simulink model "JX_Kinect_multi"  (Simulink 7.7)
settings: Solver=ode4  StartTime=0.0  StopTime=inf  FixedStep=sample_time  RelTol=1e-3
InitFcn:
  | sample_time=0.005;%0.004;%0.0025;%0.02;
  | DeltaT = 0.02;
  | g = 9.81;
  | H0 = g%0.3165;
  | Kl = 1;
  | 
  | Omega_r = 1.6;%for Horizontal reference
  | Zeta_r = 1; %for Horizontal reference
  | Omega = 1.8;%for Horizontal Control
  | Zeta = 0.5;    %for Horizontal Control
  | 
  | Omega_h_r = 2.5; %for vertical reference
  | Zeta_h_r = 0.8;  %for vertical reference
  | Omega_h = 2.7;    %for vertical control
  | Zeta_h = 0.8;         %for vertical control
  | PI=pi;
  | 
  | Mass = 1.15;
  | Acc_Max = 4;
  | Acc_Max_h = 4;
  | 
  | Max_RP = 60;
  | 
  | % for NN
  | n = 5;
  | r = 3;
  | n2 = 5;
  | NN_ST = 0.02;
  | 
  | GAMA_V = 6;
  | gama_V_e = 0.01;
  | 
  | GAMA_W = GAMA_V;
  | gama_W_e =0.01;
  | 
  | % deadzone
  | NN_Deadzone_Z = 0;
  | 
  | % inputs nomalizaton parameters
  | NN_Z_y_min = -3;
  | NN_Z_y_max = 0.5;
  | 
  | NN_Z_v_max = 8;
  | NN_Z_v_min = -NN_Z_v_max;
  | 
  | % alpha = 0.034;
  | alpha = 1;
  | % c_f = 0.0015;
  | c_f = 0.001;
  | c_y_tilt = 1*0.5;
  | 
  | %for WK paras
  | Heightcontrol = 0.08;
  | Scale_Factor=1;
  | yoffset=0;
  | 
  | load MaoBi_Oct04_2_int.mat
  | MB_Interp.time = [];
undefined symbols (not defined in the file or in its folder): DiscIntNeverNeededParam
libraries: simulink x14, dspadpt3 x6, X330_Control x4, nid_lib x2
(part 3 of 4)

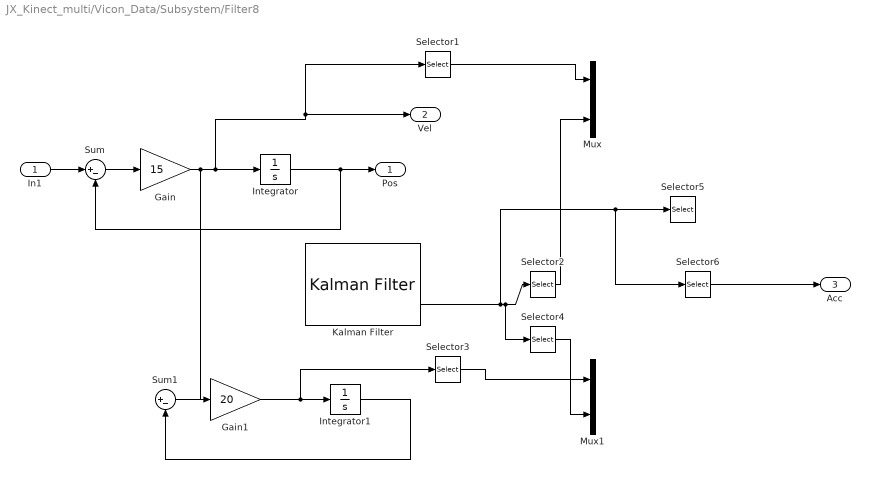
== system JX_Kinect_multi/Vicon_Data/Subsystem/Filter8 ==
  In1 : Inport
  Gain : Gain  Gain=15
  Gain1 : Gain  Gain=20
  Integrator : Integrator
  Integrator1 : Integrator
  Kalman Filter : dspadpt3/Kalman Filter  SystemSampleTime=-1  num_targets=1  sourceEnable=Always  isReset=on  X=zeros([9, 1])  P=zeros(9)  A=[1 sample_time sample_time*sample_time/2 zeros(1,6);0 1 sample_time zeros(1,6);0 0 1 zeros(1,6);0 0 0 1 sample_time sample_time*sample_time/2 0 0 0;zeros(1,4) 1 sample_time zeros(1,3);zeros(1,5) 1 zeros(1,3);zeros(1,6) 1 sample_time sample_time*sample_time/2;zeros(1,7) 1 sample_time;zeros(1,8) 1]  sourceMeasure=Specify via Dialog  H=[1 zeros(1,8); zeros(1,3) 1 zeros(1,5);zeros(1,6) 1 0 0]  Q=diag([0 0.001 0.001 0 0.001 0.001 0 0.001 0.001])  R=0.001*eye(3)  isOutputEstMeasure=on  isOutputEstState=on  isOutputEstError=off  isOutputPrdMeasure=off  isOutputPrdState=off  isOutputPrdError=off
  Mux : Mux  Inputs=2
  Mux1 : Mux  Inputs=2
  Selector1 : Selector  InputPortWidth=3  IndexOptions=Index vector (dialog)  Indices=[2]  OutputSizes=1
  Selector2 : Selector  InputPortWidth=9  IndexOptions=Index vector (dialog)  Indices=[5]  OutputSizes=1
  Selector3 : Selector  InputPortWidth=3  IndexOptions=Index vector (dialog)  Indices=[2]  OutputSizes=1
  Selector4 : Selector  InputPortWidth=9  IndexOptions=Index vector (dialog)  Indices=[6]  OutputSizes=1
  Selector5 : Selector  InputPortWidth=9  IndexOptions=Index vector (dialog)  Indices=[2 5 8]  OutputSizes=1
  Selector6 : Selector  InputPortWidth=9  IndexOptions=Index vector (dialog)  Indices=[3 6 9]  OutputSizes=1
  Sum : Sum  Inputs=|+-
  Sum1 : Sum  Inputs=|+-
  Pos : Outport
  Vel : Outport  Port=2
  Acc : Outport  Port=3
  wires:
  Selector6/1 -> Acc/1
  Selector4/1 -> Mux1/2
  Selector3/1 -> Mux1/1
  Selector2/1 -> Mux/2
  Integrator1/1 -> Sum1/2
  Gain1/1 -> Selector3/1, Integrator1/1
  Sum1/1 -> Gain1/1
  Kalman Filter/2 -> Selector6/1, Selector5/1, Selector2/1, Selector4/1
  Selector1/1 -> Mux/1
  In1/1 -> Sum/1
  Integrator/1 -> Sum/2, Pos/1
  Gain/1 -> Sum1/1, Vel/1, Selector1/1, Integrator/1
  Sum/1 -> Gain/1

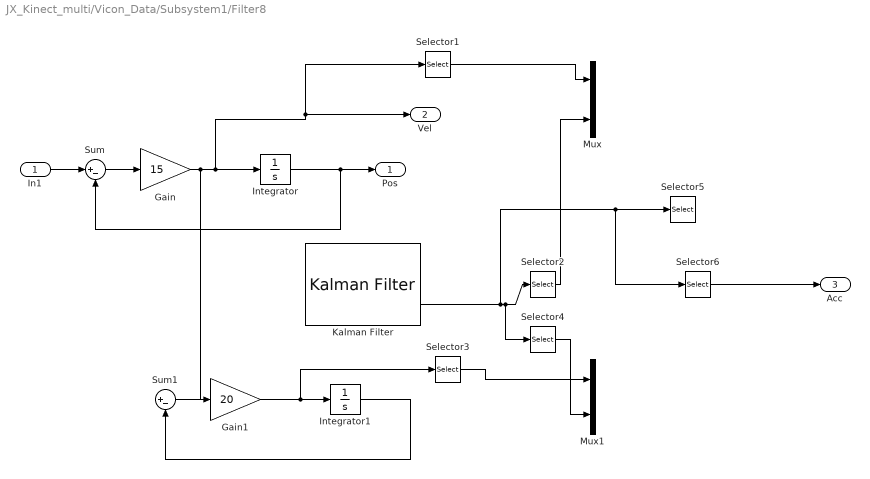
== system JX_Kinect_multi/Vicon_Data/Subsystem1/Filter8 ==
  In1 : Inport
  Gain : Gain  Gain=15
  Gain1 : Gain  Gain=20
  Integrator : Integrator
  Integrator1 : Integrator
  Kalman Filter : dspadpt3/Kalman Filter  SystemSampleTime=-1  num_targets=1  sourceEnable=Always  isReset=on  X=zeros([9, 1])  P=zeros(9)  A=[1 sample_time sample_time*sample_time/2 zeros(1,6);0 1 sample_time zeros(1,6);0 0 1 zeros(1,6);0 0 0 1 sample_time sample_time*sample_time/2 0 0 0;zeros(1,4) 1 sample_time zeros(1,3);zeros(1,5) 1 zeros(1,3);zeros(1,6) 1 sample_time sample_time*sample_time/2;zeros(1,7) 1 sample_time;zeros(1,8) 1]  sourceMeasure=Specify via Dialog  H=[1 zeros(1,8); zeros(1,3) 1 zeros(1,5);zeros(1,6) 1 0 0]  Q=diag([0 0.001 0.001 0 0.001 0.001 0 0.001 0.001])  R=0.001*eye(3)  isOutputEstMeasure=on  isOutputEstState=on  isOutputEstError=off  isOutputPrdMeasure=off  isOutputPrdState=off  isOutputPrdError=off
  Mux : Mux  Inputs=2
  Mux1 : Mux  Inputs=2
  Selector1 : Selector  InputPortWidth=3  IndexOptions=Index vector (dialog)  Indices=[2]  OutputSizes=1
  Selector2 : Selector  InputPortWidth=9  IndexOptions=Index vector (dialog)  Indices=[5]  OutputSizes=1
  Selector3 : Selector  InputPortWidth=3  IndexOptions=Index vector (dialog)  Indices=[2]  OutputSizes=1
  Selector4 : Selector  InputPortWidth=9  IndexOptions=Index vector (dialog)  Indices=[6]  OutputSizes=1
  Selector5 : Selector  InputPortWidth=9  IndexOptions=Index vector (dialog)  Indices=[2 5 8]  OutputSizes=1
  Selector6 : Selector  InputPortWidth=9  IndexOptions=Index vector (dialog)  Indices=[3 6 9]  OutputSizes=1
  Sum : Sum  Inputs=|+-
  Sum1 : Sum  Inputs=|+-
  Pos : Outport
  Vel : Outport  Port=2
  Acc : Outport  Port=3
  wires:
  Selector6/1 -> Acc/1
  Selector4/1 -> Mux1/2
  Selector3/1 -> Mux1/1
  Selector2/1 -> Mux/2
  Integrator1/1 -> Sum1/2
  Gain1/1 -> Selector3/1, Integrator1/1
  Sum1/1 -> Gain1/1
  Kalman Filter/2 -> Selector6/1, Selector5/1, Selector2/1, Selector4/1
  Selector1/1 -> Mux/1
  In1/1 -> Sum/1
  Integrator/1 -> Sum/2, Pos/1
  Gain/1 -> Sum1/1, Vel/1, Selector1/1, Integrator/1
  Sum/1 -> Gain/1

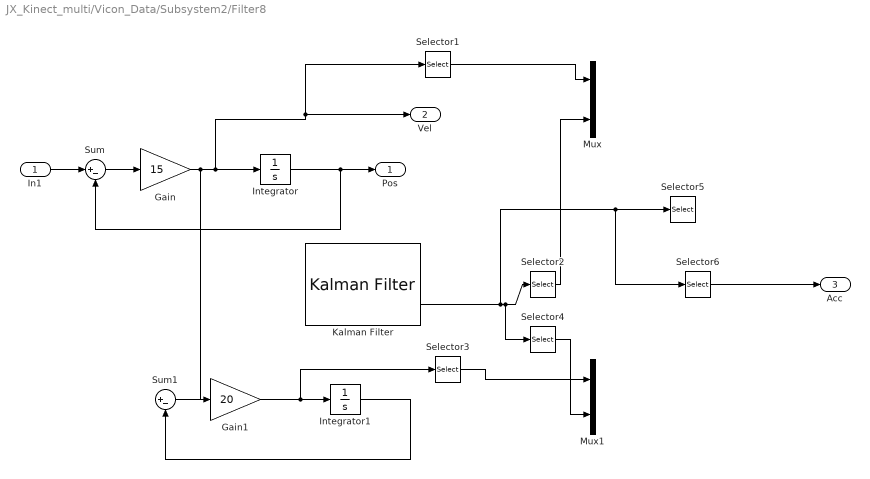
== system JX_Kinect_multi/Vicon_Data/Subsystem2/Filter8 ==
  In1 : Inport
  Gain : Gain  Gain=15
  Gain1 : Gain  Gain=20
  Integrator : Integrator
  Integrator1 : Integrator
  Kalman Filter : dspadpt3/Kalman Filter  SystemSampleTime=-1  num_targets=1  sourceEnable=Always  isReset=on  X=zeros([9, 1])  P=zeros(9)  A=[1 sample_time sample_time*sample_time/2 zeros(1,6);0 1 sample_time zeros(1,6);0 0 1 zeros(1,6);0 0 0 1 sample_time sample_time*sample_time/2 0 0 0;zeros(1,4) 1 sample_time zeros(1,3);zeros(1,5) 1 zeros(1,3);zeros(1,6) 1 sample_time sample_time*sample_time/2;zeros(1,7) 1 sample_time;zeros(1,8) 1]  sourceMeasure=Specify via Dialog  H=[1 zeros(1,8); zeros(1,3) 1 zeros(1,5);zeros(1,6) 1 0 0]  Q=diag([0 0.001 0.001 0 0.001 0.001 0 0.001 0.001])  R=0.001*eye(3)  isOutputEstMeasure=on  isOutputEstState=on  isOutputEstError=off  isOutputPrdMeasure=off  isOutputPrdState=off  isOutputPrdError=off
  Mux : Mux  Inputs=2
  Mux1 : Mux  Inputs=2
  Selector1 : Selector  InputPortWidth=3  IndexOptions=Index vector (dialog)  Indices=[2]  OutputSizes=1
  Selector2 : Selector  InputPortWidth=9  IndexOptions=Index vector (dialog)  Indices=[5]  OutputSizes=1
  Selector3 : Selector  InputPortWidth=3  IndexOptions=Index vector (dialog)  Indices=[2]  OutputSizes=1
  Selector4 : Selector  InputPortWidth=9  IndexOptions=Index vector (dialog)  Indices=[6]  OutputSizes=1
  Selector5 : Selector  InputPortWidth=9  IndexOptions=Index vector (dialog)  Indices=[2 5 8]  OutputSizes=1
  Selector6 : Selector  InputPortWidth=9  IndexOptions=Index vector (dialog)  Indices=[3 6 9]  OutputSizes=1
  Sum : Sum  Inputs=|+-
  Sum1 : Sum  Inputs=|+-
  Pos : Outport
  Vel : Outport  Port=2
  Acc : Outport  Port=3
  wires:
  Selector6/1 -> Acc/1
  Selector4/1 -> Mux1/2
  Selector3/1 -> Mux1/1
  Selector2/1 -> Mux/2
  Integrator1/1 -> Sum1/2
  Gain1/1 -> Selector3/1, Integrator1/1
  Sum1/1 -> Gain1/1
  Kalman Filter/2 -> Selector6/1, Selector5/1, Selector2/1, Selector4/1
  Selector1/1 -> Mux/1
  In1/1 -> Sum/1
  Integrator/1 -> Sum/2, Pos/1
  Gain/1 -> Sum1/1, Vel/1, Selector1/1, Integrator/1
  Sum/1 -> Gain/1

== system JX_Kinect_multi/Vicon_Data/Vicon Filter/Filter7 ==
  In1 : Inport
  Kalman Filter : dspadpt3/Kalman Filter  SystemSampleTime=-1  num_targets=1  sourceEnable=Always  isReset=on  X=zeros([12, 1])  P=zeros(12)  A=[1 sample_time sample_time*sample_time/2 zeros(1,9);0 1 sample_time zeros(1,9);0 0 1 zeros(1,9);0 0 0 1 sample_time sample_time*sample_time/2 zeros(1,6);zeros(1,4) 1 sample_time zeros(1,6);zeros(1,5) 1 zeros(1,6);zeros(1,6) 1 sample_time sample_time*sample_time/2 zeros(1,3);zeros(1,7) 1 sample_time zeros(1,3);zeros(1,8) 1 zeros(1,3);zeros(1,9) 1 sample_time sample_time*sample_time/2;zeros(1,10) 1 sample_time;zeros(1,11) 1];  sourceMeasure=Specify via Dialog  H=[1 zeros(1,11); zeros(1,3) 1 zeros(1,8);zeros(1,6) 1 zeros(1,5);zeros(1,9) 1 0 0]  Q=diag([0 0.001 0.001 0 0.001 0.001 0 0.001 0.001 0 0.001 0.001]);  R=diag([0.001 0.001 0.001 0.05])  isOutputEstMeasure=off  isOutputEstState=on  isOutputEstError=off  isOutputPrdMeasure=off  isOutputPrdState=off  isOutputPrdError=off
  Selector1 : Selector  InputPortWidth=12  IndexOptions=Index vector (dialog)  Indices=[10]  OutputSizes=1
  Selector5 : Selector  InputPortWidth=12  IndexOptions=Index vector (dialog)  Indices=[2 5 8]  OutputSizes=1
  Selector6 : Selector  InputPortWidth=12  IndexOptions=Index vector (dialog)  Indices=[3 6 9]  OutputSizes=1
  Vel : Outport
  Acc : Outport  Port=2
  Psi : Outport  Port=3
  wires:
  Selector1/1 -> Psi/1
  Selector5/1 -> Vel/1
  In1/1 -> Kalman Filter/1
  Kalman Filter/1 -> Selector1/1, Selector5/1, Selector6/1
  Selector6/1 -> Acc/1

== system JX_Kinect_multi/Vicon_Data/Vicon Filter1/Filter7 ==
  In1 : Inport
  Kalman Filter : dspadpt3/Kalman Filter  SystemSampleTime=-1  num_targets=1  sourceEnable=Always  isReset=on  X=zeros([12, 1])  P=zeros(12)  A=[1 sample_time sample_time*sample_time/2 zeros(1,9);0 1 sample_time zeros(1,9);0 0 1 zeros(1,9);0 0 0 1 sample_time sample_time*sample_time/2 zeros(1,6);zeros(1,4) 1 sample_time zeros(1,6);zeros(1,5) 1 zeros(1,6);zeros(1,6) 1 sample_time sample_time*sample_time/2 zeros(1,3);zeros(1,7) 1 sample_time zeros(1,3);zeros(1,8) 1 zeros(1,3);zeros(1,9) 1 sample_time sample_time*sample_time/2;zeros(1,10) 1 sample_time;zeros(1,11) 1];  sourceMeasure=Specify via Dialog  H=[1 zeros(1,11); zeros(1,3) 1 zeros(1,8);zeros(1,6) 1 zeros(1,5);zeros(1,9) 1 0 0]  Q=diag([0 0.001 0.001 0 0.001 0.001 0 0.001 0.001 0 0.001 0.001]);  R=diag([0.001 0.001 0.001 0.05])  isOutputEstMeasure=off  isOutputEstState=on  isOutputEstError=off  isOutputPrdMeasure=off  isOutputPrdState=off  isOutputPrdError=off
  Selector1 : Selector  InputPortWidth=12  IndexOptions=Index vector (dialog)  Indices=[10]  OutputSizes=1
  Selector5 : Selector  InputPortWidth=12  IndexOptions=Index vector (dialog)  Indices=[2 5 8]  OutputSizes=1
  Selector6 : Selector  InputPortWidth=12  IndexOptions=Index vector (dialog)  Indices=[3 6 9]  OutputSizes=1
  Vel : Outport
  Acc : Outport  Port=2
  Psi : Outport  Port=3
  wires:
  Selector1/1 -> Psi/1
  Selector5/1 -> Vel/1
  In1/1 -> Kalman Filter/1
  Kalman Filter/1 -> Selector1/1, Selector5/1, Selector6/1
  Selector6/1 -> Acc/1

== system JX_Kinect_multi/Vicon_Data/Vicon Filter2/Filter7 ==
  In1 : Inport
  Kalman Filter : dspadpt3/Kalman Filter  SystemSampleTime=-1  num_targets=1  sourceEnable=Always  isReset=on  X=zeros([12, 1])  P=zeros(12)  A=[1 sample_time sample_time*sample_time/2 zeros(1,9);0 1 sample_time zeros(1,9);0 0 1 zeros(1,9);0 0 0 1 sample_time sample_time*sample_time/2 zeros(1,6);zeros(1,4) 1 sample_time zeros(1,6);zeros(1,5) 1 zeros(1,6);zeros(1,6) 1 sample_time sample_time*sample_time/2 zeros(1,3);zeros(1,7) 1 sample_time zeros(1,3);zeros(1,8) 1 zeros(1,3);zeros(1,9) 1 sample_time sample_time*sample_time/2;zeros(1,10) 1 sample_time;zeros(1,11) 1];  sourceMeasure=Specify via Dialog  H=[1 zeros(1,11); zeros(1,3) 1 zeros(1,8);zeros(1,6) 1 zeros(1,5);zeros(1,9) 1 0 0]  Q=diag([0 0.001 0.001 0 0.001 0.001 0 0.001 0.001 0 0.001 0.001]);  R=diag([0.001 0.001 0.001 0.05])  isOutputEstMeasure=off  isOutputEstState=on  isOutputEstError=off  isOutputPrdMeasure=off  isOutputPrdState=off  isOutputPrdError=off
  Selector1 : Selector  InputPortWidth=12  IndexOptions=Index vector (dialog)  Indices=[10]  OutputSizes=1
  Selector5 : Selector  InputPortWidth=12  IndexOptions=Index vector (dialog)  Indices=[2 5 8]  OutputSizes=1
  Selector6 : Selector  InputPortWidth=12  IndexOptions=Index vector (dialog)  Indices=[3 6 9]  OutputSizes=1
  Vel : Outport
  Acc : Outport  Port=2
  Psi : Outport  Port=3
  wires:
  Selector1/1 -> Psi/1
  Selector5/1 -> Vel/1
  In1/1 -> Kalman Filter/1
  Kalman Filter/1 -> Selector1/1, Selector5/1, Selector6/1
  Selector6/1 -> Acc/1

== system JX_Kinect_multi/Kinect/Subsystem/Front or Center or Back/If Back ==
  In1 : Inport
  Action Port : ActionPort  ActionType=else
  Out1 : Outport
  wires:
  In1/1 -> Out1/1

== system JX_Kinect_multi/Kinect/Subsystem/Front or Center or Back/If Center ==
  In1 : Inport
  Action Port : ActionPort  ActionType=elseif
  Out1 : Outport
  wires:
  In1/1 -> Out1/1

== system JX_Kinect_multi/Kinect/Subsystem/Front or Center or Back/If front ==
  In1 : Inport
  Action Port : ActionPort  ActionType=then
  Out1 : Outport
  wires:
  In1/1 -> Out1/1

== system JX_Kinect_multi/Kinect/Subsystem/Up or Center or Down/Center ==
  In1 : Inport
  Action Port : ActionPort  ActionType=elseif
  Out1 : Outport
  wires:
  In1/1 -> Out1/1

== system JX_Kinect_multi/Kinect/Subsystem/Up or Center or Down/Down max ==
  In1 : Inport
  Action Port : ActionPort  ActionType=else
  Out1 : Outport
  wires:
  In1/1 -> Out1/1

== system JX_Kinect_multi/Kinect/Subsystem/Up or Center or Down/Down1 ==
  In1 : Inport
  Action Port : ActionPort  ActionType=elseif
  Out1 : Outport
  wires:
  In1/1 -> Out1/1

== system JX_Kinect_multi/Kinect/Subsystem/Up or Center or Down/Top1 ==
  In1 : Inport
  Action Port : ActionPort  ActionType=then
  Out1 : Outport
  wires:
  In1/1 -> Out1/1

== system JX_Kinect_multi/Kinect/Subsystem1/Up or Center or Down/Center ==
  In1 : Inport
  Action Port : ActionPort  ActionType=elseif
  Out1 : Outport
  wires:
  In1/1 -> Out1/1

== system JX_Kinect_multi/Kinect/Subsystem1/Up or Center or Down/Down1 ==
  In1 : Inport
  Action Port : ActionPort  ActionType=else
  Out1 : Outport
  wires:
  In1/1 -> Out1/1

== system JX_Kinect_multi/Kinect/Subsystem1/Up or Center or Down/Top1 ==
  In1 : Inport
  Action Port : ActionPort  ActionType=then
  Out1 : Outport
  wires:
  In1/1 -> Out1/1

== system JX_Kinect_multi/Vicon_Data/Raw Quad Pose from Vicon/Process Vicon Raw Data1/Flip_pi1 ==
  Angle : Inport
  Add : Sum  Inputs=-+
  Compare To Constant1 : simulink/Logic and Bit Operations/Compare To Constant  SystemSampleTime=-1  relop=>  const=pi  LogicOutDataTypeMode=uint8  ZeroCross=off
  Constant : Constant  Value=2*pi
  Data Type Duplicate : DataTypeDuplicate
  Flip_0_to_2pi : Subsystem
      mask Type: Flip zero to 2pi
      mask Description: Flips the inputs into the range zero to +2pi
      mask Help: Flips the inputs into the range zero to +2pi
      mask Display: disp('Flip_0_2pi')
  Switch : Switch  Criteria=u2 ~= 0
  Angle_Flip : Outport
  wires:
  Angle/1 -> Flip_0_to_2pi/1(Angle), Data Type Duplicate/2
  Flip_0_to_2pi/1(Angle_Flip) -> Switch/3, Compare To Constant1/1, Add/2
  Compare To Constant1/1 -> Switch/2
  Constant/1 -> Add/1
  Add/1 -> Switch/1
  Switch/1 -> Angle_Flip/1, Data Type Duplicate/1

== system JX_Kinect_multi/Vicon_Data/Raw Quad Pose from Vicon/Process Vicon Raw Data2/Flip_pi1 ==
  Angle : Inport
  Add : Sum  Inputs=-+
  Compare To Constant1 : simulink/Logic and Bit Operations/Compare To Constant  SystemSampleTime=-1  relop=>  const=pi  LogicOutDataTypeMode=uint8  ZeroCross=off
  Constant : Constant  Value=2*pi
  Data Type Duplicate : DataTypeDuplicate
  Flip_0_to_2pi : Subsystem
      mask Type: Flip zero to 2pi
      mask Description: Flips the inputs into the range zero to +2pi
      mask Help: Flips the inputs into the range zero to +2pi
      mask Display: disp('Flip_0_2pi')
  Switch : Switch  Criteria=u2 ~= 0
  Angle_Flip : Outport
  wires:
  Switch/1 -> Data Type Duplicate/1, Angle_Flip/1
  Add/1 -> Switch/1
  Constant/1 -> Add/1
  Compare To Constant1/1 -> Switch/2
  Flip_0_to_2pi/1(Angle_Flip) -> Add/2, Compare To Constant1/1, Switch/3
  Angle/1 -> Data Type Duplicate/2, Flip_0_to_2pi/1(Angle)

== system JX_Kinect_multi/Vicon_Data/Raw Quad Pose from Vicon/Process Vicon Raw Data3/Flip_pi1 ==
  Angle : Inport
  Add : Sum  Inputs=-+
  Compare To Constant1 : simulink/Logic and Bit Operations/Compare To Constant  SystemSampleTime=-1  relop=>  const=pi  LogicOutDataTypeMode=uint8  ZeroCross=off
  Constant : Constant  Value=2*pi
  Data Type Duplicate : DataTypeDuplicate
  Flip_0_to_2pi : Subsystem
      mask Type: Flip zero to 2pi
      mask Description: Flips the inputs into the range zero to +2pi
      mask Help: Flips the inputs into the range zero to +2pi
      mask Display: disp('Flip_0_2pi')
  Switch : Switch  Criteria=u2 ~= 0
  Angle_Flip : Outport
  wires:
  Angle/1 -> Flip_0_to_2pi/1(Angle), Data Type Duplicate/2
  Flip_0_to_2pi/1(Angle_Flip) -> Switch/3, Compare To Constant1/1, Add/2
  Compare To Constant1/1 -> Switch/2
  Constant/1 -> Add/1
  Add/1 -> Switch/1
  Switch/1 -> Angle_Flip/1, Data Type Duplicate/1

== system JX_Kinect_multi/Vicon_Data/Raw Quad Pose from Vicon/Process Vicon Raw Data4/Flip_pi1 ==
  Angle : Inport
  Add : Sum  Inputs=-+
  Compare To Constant1 : simulink/Logic and Bit Operations/Compare To Constant  SystemSampleTime=-1  relop=>  const=pi  LogicOutDataTypeMode=uint8  ZeroCross=off
  Constant : Constant  Value=2*pi
  Data Type Duplicate : DataTypeDuplicate
  Flip_0_to_2pi : Subsystem
      mask Type: Flip zero to 2pi
      mask Description: Flips the inputs into the range zero to +2pi
      mask Help: Flips the inputs into the range zero to +2pi
      mask Display: disp('Flip_0_2pi')
  Switch : Switch  Criteria=u2 ~= 0
  Angle_Flip : Outport
  wires:
  Switch/1 -> Data Type Duplicate/1, Angle_Flip/1
  Add/1 -> Switch/1
  Constant/1 -> Add/1
  Compare To Constant1/1 -> Switch/2
  Flip_0_to_2pi/1(Angle_Flip) -> Add/2, Compare To Constant1/1, Switch/3
  Angle/1 -> Data Type Duplicate/2, Flip_0_to_2pi/1(Angle)

== system JX_Kinect_multi/Vicon_Data/Raw Quad Pose from Vicon/Process Vicon Raw Data6/Flip_pi1 ==
  Angle : Inport
  Add : Sum  Inputs=-+
  Compare To Constant1 : simulink/Logic and Bit Operations/Compare To Constant  SystemSampleTime=-1  relop=>  const=pi  LogicOutDataTypeMode=uint8  ZeroCross=off
  Constant : Constant  Value=2*pi
  Data Type Duplicate : DataTypeDuplicate
  Flip_0_to_2pi : Subsystem
      mask Type: Flip zero to 2pi
      mask Description: Flips the inputs into the range zero to +2pi
      mask Help: Flips the inputs into the range zero to +2pi
      mask Display: disp('Flip_0_2pi')
  Switch : Switch  Criteria=u2 ~= 0
  Angle_Flip : Outport
  wires:
  Angle/1 -> Flip_0_to_2pi/1(Angle), Data Type Duplicate/2
  Flip_0_to_2pi/1(Angle_Flip) -> Switch/3, Compare To Constant1/1, Add/2
  Compare To Constant1/1 -> Switch/2
  Constant/1 -> Add/1
  Add/1 -> Switch/1
  Switch/1 -> Angle_Flip/1, Data Type Duplicate/1

== system JX_Kinect_multi/Vicon_Data/Raw Quad Pose from Vicon/Process Vicon Raw Data7/Flip_pi1 ==
  Angle : Inport
  Add : Sum  Inputs=-+
  Compare To Constant1 : simulink/Logic and Bit Operations/Compare To Constant  SystemSampleTime=-1  relop=>  const=pi  LogicOutDataTypeMode=uint8  ZeroCross=off
  Constant : Constant  Value=2*pi
  Data Type Duplicate : DataTypeDuplicate
  Flip_0_to_2pi : Subsystem
      mask Type: Flip zero to 2pi
      mask Description: Flips the inputs into the range zero to +2pi
      mask Help: Flips the inputs into the range zero to +2pi
      mask Display: disp('Flip_0_2pi')
  Switch : Switch  Criteria=u2 ~= 0
  Angle_Flip : Outport
  wires:
  Switch/1 -> Data Type Duplicate/1, Angle_Flip/1
  Add/1 -> Switch/1
  Constant/1 -> Add/1
  Compare To Constant1/1 -> Switch/2
  Flip_0_to_2pi/1(Angle_Flip) -> Add/2, Compare To Constant1/1, Switch/3
  Angle/1 -> Data Type Duplicate/2, Flip_0_to_2pi/1(Angle)

== system JX_Kinect_multi/Vicon_Data/Raw Quad Pose from Vicon/Process Vicon Raw Data1/Flip_pi1/Flip_0_to_2pi ==
  Angle : Inport
  Add : Sum
  Compare To Constant1 : simulink/Logic and Bit Operations/Compare To Constant  SystemSampleTime=-1  relop=<  const=0  LogicOutDataTypeMode=uint8  ZeroCross=off
  Constant : Constant  Value=2*pi
  Data Type Duplicate : DataTypeDuplicate
  Flip_2pi : Subsystem
      mask Type: Flip -2pi to 2pi
      mask Description: Flips the inputs into the range -2pi to +2pi
      mask Help: Flips the inputs into the range -2pi to +2pi
      mask Display: disp('Flip_2pi')
  Switch : Switch  Criteria=u2 ~= 0
  Angle_Flip : Outport
  wires:
  Flip_2pi/1(Angle_Flip) -> Compare To Constant1/1, Add/2, Switch/3
  Compare To Constant1/1 -> Switch/2
  Constant/1 -> Add/1
  Add/1 -> Switch/1
  Angle/1 -> Flip_2pi/1(Angle), Data Type Duplicate/2
  Switch/1 -> Angle_Flip/1, Data Type Duplicate/1

== system JX_Kinect_multi/Vicon_Data/Raw Quad Pose from Vicon/Process Vicon Raw Data2/Flip_pi1/Flip_0_to_2pi ==
  Angle : Inport
  Add : Sum
  Compare To Constant1 : simulink/Logic and Bit Operations/Compare To Constant  SystemSampleTime=-1  relop=<  const=0  LogicOutDataTypeMode=uint8  ZeroCross=off
  Constant : Constant  Value=2*pi
  Data Type Duplicate : DataTypeDuplicate
  Flip_2pi : Subsystem
      mask Type: Flip -2pi to 2pi
      mask Description: Flips the inputs into the range -2pi to +2pi
      mask Help: Flips the inputs into the range -2pi to +2pi
      mask Display: disp('Flip_2pi')
  Switch : Switch  Criteria=u2 ~= 0
  Angle_Flip : Outport
  wires:
  Switch/1 -> Data Type Duplicate/1, Angle_Flip/1
  Angle/1 -> Data Type Duplicate/2, Flip_2pi/1(Angle)
  Add/1 -> Switch/1
  Constant/1 -> Add/1
  Compare To Constant1/1 -> Switch/2
  Flip_2pi/1(Angle_Flip) -> Switch/3, Add/2, Compare To Constant1/1

== system JX_Kinect_multi/Vicon_Data/Raw Quad Pose from Vicon/Process Vicon Raw Data3/Flip_pi1/Flip_0_to_2pi ==
  Angle : Inport
  Add : Sum
  Compare To Constant1 : simulink/Logic and Bit Operations/Compare To Constant  SystemSampleTime=-1  relop=<  const=0  LogicOutDataTypeMode=uint8  ZeroCross=off
  Constant : Constant  Value=2*pi
  Data Type Duplicate : DataTypeDuplicate
  Flip_2pi : Subsystem
      mask Type: Flip -2pi to 2pi
      mask Description: Flips the inputs into the range -2pi to +2pi
      mask Help: Flips the inputs into the range -2pi to +2pi
      mask Display: disp('Flip_2pi')
  Switch : Switch  Criteria=u2 ~= 0
  Angle_Flip : Outport
  wires:
  Flip_2pi/1(Angle_Flip) -> Compare To Constant1/1, Add/2, Switch/3
  Compare To Constant1/1 -> Switch/2
  Constant/1 -> Add/1
  Add/1 -> Switch/1
  Angle/1 -> Flip_2pi/1(Angle), Data Type Duplicate/2
  Switch/1 -> Angle_Flip/1, Data Type Duplicate/1

== system JX_Kinect_multi/Vicon_Data/Raw Quad Pose from Vicon/Process Vicon Raw Data4/Flip_pi1/Flip_0_to_2pi ==
  Angle : Inport
  Add : Sum
  Compare To Constant1 : simulink/Logic and Bit Operations/Compare To Constant  SystemSampleTime=-1  relop=<  const=0  LogicOutDataTypeMode=uint8  ZeroCross=off
  Constant : Constant  Value=2*pi
  Data Type Duplicate : DataTypeDuplicate
  Flip_2pi : Subsystem
      mask Type: Flip -2pi to 2pi
      mask Description: Flips the inputs into the range -2pi to +2pi
      mask Help: Flips the inputs into the range -2pi to +2pi
      mask Display: disp('Flip_2pi')
  Switch : Switch  Criteria=u2 ~= 0
  Angle_Flip : Outport
  wires:
  Switch/1 -> Data Type Duplicate/1, Angle_Flip/1
  Angle/1 -> Data Type Duplicate/2, Flip_2pi/1(Angle)
  Add/1 -> Switch/1
  Constant/1 -> Add/1
  Compare To Constant1/1 -> Switch/2
  Flip_2pi/1(Angle_Flip) -> Switch/3, Add/2, Compare To Constant1/1

== system JX_Kinect_multi/Vicon_Data/Raw Quad Pose from Vicon/Process Vicon Raw Data6/Flip_pi1/Flip_0_to_2pi ==
  Angle : Inport
  Add : Sum
  Compare To Constant1 : simulink/Logic and Bit Operations/Compare To Constant  SystemSampleTime=-1  relop=<  const=0  LogicOutDataTypeMode=uint8  ZeroCross=off
  Constant : Constant  Value=2*pi
  Data Type Duplicate : DataTypeDuplicate
  Flip_2pi : Subsystem
      mask Type: Flip -2pi to 2pi
      mask Description: Flips the inputs into the range -2pi to +2pi
      mask Help: Flips the inputs into the range -2pi to +2pi
      mask Display: disp('Flip_2pi')
  Switch : Switch  Criteria=u2 ~= 0
  Angle_Flip : Outport
  wires:
  Flip_2pi/1(Angle_Flip) -> Compare To Constant1/1, Add/2, Switch/3
  Compare To Constant1/1 -> Switch/2
  Constant/1 -> Add/1
  Add/1 -> Switch/1
  Angle/1 -> Flip_2pi/1(Angle), Data Type Duplicate/2
  Switch/1 -> Angle_Flip/1, Data Type Duplicate/1

== system JX_Kinect_multi/Vicon_Data/Raw Quad Pose from Vicon/Process Vicon Raw Data7/Flip_pi1/Flip_0_to_2pi ==
  Angle : Inport
  Add : Sum
  Compare To Constant1 : simulink/Logic and Bit Operations/Compare To Constant  SystemSampleTime=-1  relop=<  const=0  LogicOutDataTypeMode=uint8  ZeroCross=off
  Constant : Constant  Value=2*pi
  Data Type Duplicate : DataTypeDuplicate
  Flip_2pi : Subsystem
      mask Type: Flip -2pi to 2pi
      mask Description: Flips the inputs into the range -2pi to +2pi
      mask Help: Flips the inputs into the range -2pi to +2pi
      mask Display: disp('Flip_2pi')
  Switch : Switch  Criteria=u2 ~= 0
  Angle_Flip : Outport
  wires:
  Switch/1 -> Data Type Duplicate/1, Angle_Flip/1
  Angle/1 -> Data Type Duplicate/2, Flip_2pi/1(Angle)
  Add/1 -> Switch/1
  Constant/1 -> Add/1
  Compare To Constant1/1 -> Switch/2
  Flip_2pi/1(Angle_Flip) -> Switch/3, Add/2, Compare To Constant1/1

== system JX_Kinect_multi/Vicon_Data/Raw Quad Pose from Vicon/Process Vicon Raw Data1/Flip_pi1/Flip_0_to_2pi/Flip_2pi ==
  Angle : Inport
  Bias : Bias  Bias=-2*pi
  Constant : Constant  Value=2*pi
  Data Type Duplicate : DataTypeDuplicate
  Modulo : Math  Operator=mod  SaturateOnIntegerOverflow=on
  Sign1 : Signum
  Switch : Switch
  Angle_Flip : Outport
  wires:
  Angle/1 -> Modulo/1, Sign1/1, Data Type Duplicate/1
  Constant/1 -> Modulo/2
  Modulo/1 -> Bias/1, Switch/1
  Sign1/1 -> Switch/2
  Bias/1 -> Switch/3
  Switch/1 -> Angle_Flip/1, Data Type Duplicate/2

== system JX_Kinect_multi/Vicon_Data/Raw Quad Pose from Vicon/Process Vicon Raw Data2/Flip_pi1/Flip_0_to_2pi/Flip_2pi ==
  Angle : Inport
  Bias : Bias  Bias=-2*pi
  Constant : Constant  Value=2*pi
  Data Type Duplicate : DataTypeDuplicate
  Modulo : Math  Operator=mod  SaturateOnIntegerOverflow=on
  Sign1 : Signum
  Switch : Switch
  Angle_Flip : Outport
  wires:
  Switch/1 -> Data Type Duplicate/2, Angle_Flip/1
  Bias/1 -> Switch/3
  Sign1/1 -> Switch/2
  Modulo/1 -> Switch/1, Bias/1
  Constant/1 -> Modulo/2
  Angle/1 -> Data Type Duplicate/1, Sign1/1, Modulo/1

== system JX_Kinect_multi/Vicon_Data/Raw Quad Pose from Vicon/Process Vicon Raw Data3/Flip_pi1/Flip_0_to_2pi/Flip_2pi ==
  Angle : Inport
  Bias : Bias  Bias=-2*pi
  Constant : Constant  Value=2*pi
  Data Type Duplicate : DataTypeDuplicate
  Modulo : Math  Operator=mod  SaturateOnIntegerOverflow=on
  Sign1 : Signum
  Switch : Switch
  Angle_Flip : Outport
  wires:
  Angle/1 -> Modulo/1, Sign1/1, Data Type Duplicate/1
  Constant/1 -> Modulo/2
  Modulo/1 -> Bias/1, Switch/1
  Sign1/1 -> Switch/2
  Bias/1 -> Switch/3
  Switch/1 -> Angle_Flip/1, Data Type Duplicate/2

== system JX_Kinect_multi/Vicon_Data/Raw Quad Pose from Vicon/Process Vicon Raw Data4/Flip_pi1/Flip_0_to_2pi/Flip_2pi ==
  Angle : Inport
  Bias : Bias  Bias=-2*pi
  Constant : Constant  Value=2*pi
  Data Type Duplicate : DataTypeDuplicate
  Modulo : Math  Operator=mod  SaturateOnIntegerOverflow=on
  Sign1 : Signum
  Switch : Switch
  Angle_Flip : Outport
  wires:
  Switch/1 -> Data Type Duplicate/2, Angle_Flip/1
  Bias/1 -> Switch/3
  Sign1/1 -> Switch/2
  Modulo/1 -> Switch/1, Bias/1
  Constant/1 -> Modulo/2
  Angle/1 -> Data Type Duplicate/1, Sign1/1, Modulo/1

== system JX_Kinect_multi/Vicon_Data/Raw Quad Pose from Vicon/Process Vicon Raw Data6/Flip_pi1/Flip_0_to_2pi/Flip_2pi ==
  Angle : Inport
  Bias : Bias  Bias=-2*pi
  Constant : Constant  Value=2*pi
  Data Type Duplicate : DataTypeDuplicate
  Modulo : Math  Operator=mod  SaturateOnIntegerOverflow=on
  Sign1 : Signum
  Switch : Switch
  Angle_Flip : Outport
  wires:
  Angle/1 -> Modulo/1, Sign1/1, Data Type Duplicate/1
  Constant/1 -> Modulo/2
  Modulo/1 -> Bias/1, Switch/1
  Sign1/1 -> Switch/2
  Bias/1 -> Switch/3
  Switch/1 -> Angle_Flip/1, Data Type Duplicate/2

== system JX_Kinect_multi/Vicon_Data/Raw Quad Pose from Vicon/Process Vicon Raw Data7/Flip_pi1/Flip_0_to_2pi/Flip_2pi ==
  Angle : Inport
  Bias : Bias  Bias=-2*pi
  Constant : Constant  Value=2*pi
  Data Type Duplicate : DataTypeDuplicate
  Modulo : Math  Operator=mod  SaturateOnIntegerOverflow=on
  Sign1 : Signum
  Switch : Switch
  Angle_Flip : Outport
  wires:
  Switch/1 -> Data Type Duplicate/2, Angle_Flip/1
  Bias/1 -> Switch/3
  Sign1/1 -> Switch/2
  Modulo/1 -> Switch/1, Bias/1
  Constant/1 -> Modulo/2
  Angle/1 -> Data Type Duplicate/1, Sign1/1, Modulo/1

== matlab function UAV1/Yaw Controller/MATLAB Function ==
  data: u input double; y output double
function y = fcn(u)
%#codegen
y = u;
if y > pi    
    y = y - 2*pi;
elseif y < -pi
        y = y + 2*pi;
end

== stateflow chart UAV2/Trajectory Logic/UAV SF ==
  state Landing
    state Descending
      en:PosDesired = Pos;
      du:PosDesired[2] = (0.1- PosDesired[2])*1*DeltaT + PosDesired[2] ;
    state CutThrottle
      en: PWM=1600;
      du:HoverThrottle = (0.0- HoverThrottle)*3*DeltaT + HoverThrottle ;
    (default) -> Descending
    Descending -> CutThrottle : [Pos[2] >(0.0 -0.1)]
  state AirBorne
    state TakeOff
      du:HoverThrottle = (H0 - HoverThrottle)*3*DeltaT + HoverThrottle ;
    state Kinect
      state Initialise
        en:
        PosDesired[0]=1.5, PosDesired[1]=-0,PosDesired[2]= -1.5,PosDesired[3]=0;
        LeftRight = 0;
        UpDown = 0;
        FrontBack = 0;
        Toggle = 1;
        ClawStatus = 1;
        Rotation = 0;
        PWM = 1690;
        LXC=0; LYC=0; LZC=0; RXYC=0; safechecker = 2;
      state UpdateQuad
        en:
        PosDesired[0]=1.5+LeftRight, PosDesired[1]=0+FrontBack,PosDesired[2]= -1.5+UpDown,PosDesired[3] = 0+Rotation;
        LHRH = 0;
        XYZchecker=0;
      state KinectTrack
        state CheckLEFTZ
          state ZCenter
            en:
            UpDown=UpDown+0;
            LZC=0;
            LHRH = 3;
          state ZDown
            en:
            UpDown=UpDown+0.02;
            LHRH = 3;
          state ZUp
            en:
            UpDown=UpDown-0.02;
            LHRH = 3;
          (junction 65) -> ZUp [order 3] : [LeftHand[2]==1]
          (junction 65) -> ZDown [order 1] : [LeftHand[2]== -1]
          (junction 65) -> ZCenter [order 2] : [LeftHand[2]==0]
          (default) -> (junction 65)
        state CheckLEFTX
          state XLeft
            en:
            LeftRight=LeftRight-0.02;
            LHRH=1;
          state XRight
            en:
            LeftRight=LeftRight+0.02;
            LHRH=1;
          state XCenter
            en:
            LeftRight=LeftRight+0;
            LXC=0;
            LHRH=1;
          (junction 63) -> XRight [order 1] : [LeftHand[0]== -1]
          (default) -> (junction 63)
          (junction 63) -> XLeft [order 3] : [LeftHand[0]==1]
          (junction 63) -> XCenter [order 2] : [LeftHand[0]==0]
        state CheckRIGHTXY
          state ToggleOpen
            en:
            ClawStatus=1;
            Toggle=2;
            LHRH=4;
          state ToggleClose
            en:
            ClawStatus=0;
            Toggle=2;
            LHRH=4;
          state RightHanddown
            en:
            Toggle=1;
            LHRH = 4;
          state ContinuousHandUp
            en:
            LHRH=4;
          state Heading
            state Clockwise
              en:
              Rotation=Rotation+0.01;
              Toggle=1;
              LHRH=4;
            state Neutral
              en:
              Rotation = Rotation +0;
              RXYC=0;
              Toggle=1;
              LHRH = 4;
            state AntiClockwise
              en:
              Rotation = Rotation - 0.01;
              Toggle=1;
              LHRH = 4;
            (default) -> (junction 73)
            (junction 73) -> Clockwise [order 3] : [RightHand[1]==1]
            (junction 73) -> AntiClockwise [order 1] : [RightHand[1]==-1]
            (junction 73) -> Neutral [order 2] : [RightHand[1]==0]
          (default) -> (junction 71)
          (junction 71) -> (junction 78) [order 3] : [RightHand[0]==1]
          (junction 71) -> RightHanddown [order 2] : [RightHand[0]== -1]
          (junction 71) -> Heading [order 1] : [RightHand[0]==0]
          (junction 78) -> ContinuousHandUp [order 1] : [Toggle==2]
          (junction 77) -> ToggleClose [order 1] : [ClawStatus==1]
          (junction 78) -> (junction 77) [order 2] : [Toggle==1]
          (junction 77) -> ToggleOpen [order 2] : [ClawStatus==0]
        state CLAW
          state OpenMax
            en:
            PWM = 1690;
            LHRH = 5;
          state CloseMax
            en:
            PWM = 1200;
            LHRH = 5;
          state OpenClaw
            en:
            PWM = PWM+100;
            LHRH = 5;
          state CloseClaw
            en:
            PWM = PWM-100;
            LHRH = 5;
          (junction 75) -> (junction 72) [order 1] : [ClawStatus==0]
          (junction 75) -> (junction 74) [order 2] : [ClawStatus==1]
          (junction 74) -> OpenMax [order 1] : [PWM>=1680]
          (junction 74) -> OpenClaw [order 2] : [PWM<1680]
          (junction 72) -> CloseClaw [order 2] : [PWM>1180]
          (junction 72) -> CloseMax [order 1] : [PWM<=1180]
          (default) -> (junction 75)
        state CheckLEFTY
          state YCenter
            en:
            FrontBack=FrontBack+0;
            LYC=0;
            LHRH = 2;
          state YFront
            en:
            FrontBack=FrontBack-0.02;
            LHRH = 2;
          state YBack
            en:
            FrontBack=FrontBack+0.02;
            LHRH = 2;
          (default) -> (junction 64)
          (junction 64) -> YFront [order 3] : [LeftHand[1]==1]
          (junction 64) -> YCenter [order 2] : [LeftHand[1]==0]
          (junction 64) -> YBack [order 1] : [LeftHand[1]== -1]
        CheckLEFTX -> CheckLEFTY : [(LHRH==1)]
        CheckLEFTY -> CheckLEFTZ : [(LHRH==2)]
        (junction 69) -> CheckLEFTX [order 2] : [LeftHand[2]~= -2]
        CheckLEFTZ -> CheckRIGHTXY : [(LHRH==3)]
        (junction 69) -> CheckRIGHTXY [order 1] : [LeftHand[2]== -2]
        CheckRIGHTXY -> CLAW : [LHRH ==4]
      state Constraint
        state PositionConstraint
          state Xpositive
            en:
            LeftRight=2;
          state Xnegative
            en:
            LeftRight=1;
          state Ypositive
            en:
            FrontBack=2;
          state Ynegative
            en:
            FrontBack=-2;
          state Zpositive
            en:
            UpDown=0.78;
          state Znegative
            en:
            UpDown=-1;
          state RotateACW
            en:
            Rotation=-3.1;
          state RotateCW
            en:
            Rotation=3.1;
          state Contained
            en:
            LHRH = 7;
          (junction 66) -> Contained [order 1] : [Rotation>=-3.1]
          Znegative -> (junction 76)
          (default) -> (junction 68)
          (junction 68) -> Xpositive [order 2] : [LeftRight>2]
          (junction 67) -> Xnegative [order 2] : [LeftRight<1]
          (junction 81) -> Ypositive [order 2] : [FrontBack>2]
          (junction 80) -> Ynegative [order 2] : [FrontBack<-2]
          (junction 79) -> Zpositive [order 2] : [UpDown>0.78]
          Xnegative -> (junction 81)
          (junction 79) -> (junction 70) [order 1] : [UpDown<=0.78]
          Ypositive -> (junction 80)
          (junction 80) -> (junction 79) [order 1] : [FrontBack>=-2]
          (junction 70) -> (junction 76) [order 1] : [UpDown>=-1]
          RotateACW -> Contained
          RotateCW -> (junction 66)
          (junction 66) -> RotateACW [order 2] : [Rotation<-3.1]
          (junction 76) -> (junction 66) [order 1] : [Rotation<=3.1]
          (junction 76) -> RotateCW [order 2] : [Rotation>3.1]
          Ynegative -> (junction 79)
          Zpositive -> (junction 70)
          (junction 70) -> Znegative [order 2] : [UpDown<-1]
          (junction 68) -> (junction 67) [order 1] : [LeftRight<=2]
          Xpositive -> (junction 67)
          (junction 67) -> (junction 81) [order 1] : [LeftRight>=1]
          (junction 81) -> (junction 80) [order 1] : [FrontBack<=2]
        state ALLGreen
          en:
          LHRH = 7;
        (junction 82) -> PositionConstraint [order 2] : [(LeftRight > 2)|(LeftRight<1)|(FrontBack>2)|(FrontBack<-2)|(UpDown>0.78)|(UpDown<-1)|(Rotation>3.1)|(Rotation<-3.1)]
        (junction 82) -> ALLGreen [order 1] : [(LeftRight<=2)&(LeftRight>=1)&(FrontBack<=2)&(FrontBack>=-2)&(UpDown<=0.78)&(UpDown>=-1)&(Rotation<=3.1)&(Rotation>=-3.1)]
        PositionConstraint -> ALLGreen : [(LeftRight<=2)&(LeftRight>=1)&(FrontBack<=2)&(FrontBack>=-2)&(UpDown<=0.78)&(UpDown>=-1)&(Rotation<=3.1)&(Rotation>=-3.1)]
        (default) -> (junction 82)
      state CheckKinect
        en:
        PosDesired[0]=1.5+LeftRight, PosDesired[1]=0+FrontBack,PosDesired[2]= -1.5+UpDown,PosDesired[3] = 0+Rotation;
      KinectTrack -> UpdateQuad [order 1] : [KinectTracking==0]
      (default) -> KinectTrack [order 1] : [KinectTracking==1]
      KinectTrack -> Constraint [order 2] : [(LHRH==5)]
      (default) -> Initialise [order 2]
      Initialise -> UpdateQuad : after (3,sec)
      Constraint -> UpdateQuad : [LHRH==7]
      UpdateQuad -> CheckKinect : [KinectTracking~=1]
      CheckKinect -> UpdateQuad : after (0.2,sec)
    state Safety
      state Descent1
        descentrate=descentrate+0.02;
      state Descent
        en:PosDesired[0] = PerchPos[0]; PosDesired[1] = PerchPos[1];PosDesired[2] = PerchPos[2]-0.50+descentrate;
      state Prelanding
        en:PosDesired[0] = PerchPos[0]; PosDesired[1] = PerchPos[1];PosDesired[2] = PerchPos[2]-0.8 ;
        descentrate=0;
      state SafyHover
        en:PosDesired = Pos; PosDesired[2]= -1.5;
      (default) -> SafyHover
      Descent1 -> Descent : after (0.5,sec)
      Descent -> Descent1 [order 2] : [PerchError < 0.02]
      Descent -> Prelanding [order 1] : after (5,sec)
      Prelanding -> Descent : [PerchError < 0.01]
      SafyHover -> Prelanding : after (3, sec)
    (default) -> TakeOff : {PosDesired = Pos;  PosDesired[2] =-1.2;}
    TakeOff -> Kinect [order 1] : after (7,sec)
    TakeOff -> Safety [order 2] : [RC[5] > 0.5]
    Kinect -> Safety : [RC[5] > 0.5]
  (default) -> Landing : {HoverThrottle = 0;}
  AirBorne -> Landing : [RC[6] < -0.5]
  Landing -> AirBorne : [RC[6] > 0.5]
  data: PosDesired output double size=4; HoverThrottle output double size=1; Mode output uint8 size=1; RC input double size=8; Pos input double size=4; PerchPos input double size=4; DeltaT parameter double size=1; H0 parameter double size=1; Kl parameter double size=1; VelCmd local double size=2 =0; PWM output double; PerchError input double; PI parameter double size=1; descentrate local double; LeftHand input double; KinectTracking input double; UpDown local double; FrontBack local double; XYZchecker local double; RightHand input double; ClawStatus local double; LHRH local double; Rotation local double; LeftRight local double; LXC local double; LYC local double; LZC local double; RXYC local double; safechecker local double; Toggle local double

== stateflow chart UAV1/Trajectory Logic/UAV SF ==
  state Landing
    state Descending
      en:PosDesired = Pos;
      du:PosDesired[2] = (0.1- PosDesired[2])*1*DeltaT + PosDesired[2] ;
    state CutThrottle
      en: PWM=1600;
      du:HoverThrottle = (0.0- HoverThrottle)*3*DeltaT + HoverThrottle ;
    (default) -> Descending
    Descending -> CutThrottle : [Pos[2] >(0.0 -0.1)]
  state AirBorne
    state TakeOff
      du:HoverThrottle = (H0 - HoverThrottle)*3*DeltaT + HoverThrottle ;
    state Kinect
      state Initialise
        en:
        PosDesired[0]=-1.5, PosDesired[1]=0,PosDesired[2]= -1.5,PosDesired[3]=0;
        LeftRight = 0;
        UpDown = 0;
        FrontBack = 0;
        Toggle = 1;
        ClawStatus = 1;
        Rotation = 0;
        PWM = 1690;
        LXC=0; LYC=0; LZC=0; RXYC=0; safechecker = 2;
      state UpdateQuad
        en:
        PosDesired[0]=-1.5+LeftRight, PosDesired[1]=0+FrontBack,PosDesired[2]= -1.5+UpDown,PosDesired[3] = 0+Rotation;
        LHRH = 0;
        XYZchecker=0;
      state KinectTrack
        state CheckLEFTZ
          state ZCenter
            en:
            UpDown=UpDown+0;
            LZC=0;
            LHRH = 3;
          state ZDown
            en:
            UpDown=UpDown+0.02;
            LHRH = 3;
          state ZUp
            en:
            UpDown=UpDown-0.02;
            LHRH = 3;
          (junction 259) -> ZUp [order 3] : [LeftHand[2]==1]
          (junction 259) -> ZDown [order 1] : [LeftHand[2]== -1]
          (junction 259) -> ZCenter [order 2] : [LeftHand[2]==0]
          (default) -> (junction 259)
        state CheckLEFTX
          state XLeft
            en:
            LeftRight=LeftRight-0.02;
            LHRH=1;
          state XRight
            en:
            LeftRight=LeftRight+0.02;
            LHRH=1;
          state XCenter
            en:
            LeftRight=LeftRight+0;
            LXC=0;
            LHRH=1;
          (junction 257) -> XRight [order 1] : [LeftHand[0]== -1]
          (default) -> (junction 257)
          (junction 257) -> XLeft [order 3] : [LeftHand[0]==1]
          (junction 257) -> XCenter [order 2] : [LeftHand[0]==0]
        state CheckRIGHTXY
          state ToggleOpen
            en:
            ClawStatus=1;
            Toggle=2;
            LHRH=4;
          state ToggleClose
            en:
            ClawStatus=0;
            Toggle=2;
            LHRH=4;
          state RightHanddown
            en:
            Toggle=1;
            LHRH = 4;
          state ContinuousHandUp
            en:
            LHRH=4;
          state Heading
            state Clockwise
              en:
              Rotation=Rotation+0.01;
              Toggle=1;
              LHRH=4;
            state Neutral
              en:
              Rotation = Rotation +0;
              RXYC=0;
              Toggle=1;
              LHRH = 4;
            state AntiClockwise
              en:
              Rotation = Rotation - 0.01;
              Toggle=1;
              LHRH = 4;
            (default) -> (junction 267)
            (junction 267) -> Clockwise [order 3] : [RightHand[1]==1]
            (junction 267) -> AntiClockwise [order 1] : [RightHand[1]==-1]
            (junction 267) -> Neutral [order 2] : [RightHand[1]==0]
          (default) -> (junction 265)
          (junction 265) -> (junction 272) [order 3] : [RightHand[0]==1]
          (junction 265) -> RightHanddown [order 2] : [RightHand[0]== -1]
          (junction 265) -> Heading [order 1] : [RightHand[0]==0]
          (junction 272) -> ContinuousHandUp [order 1] : [Toggle==2]
          (junction 271) -> ToggleClose [order 1] : [ClawStatus==1]
          (junction 272) -> (junction 271) [order 2] : [Toggle==1]
          (junction 271) -> ToggleOpen [order 2] : [ClawStatus==0]
        state CLAW
          state OpenMax
            en:
            PWM = 1690;
            LHRH = 5;
          state CloseMax
            en:
            PWM = 1200;
            LHRH = 5;
          state OpenClaw
            en:
            PWM = PWM+100;
            LHRH = 5;
          state CloseClaw
            en:
            PWM = PWM-100;
            LHRH = 5;
          (junction 269) -> (junction 266) [order 1] : [ClawStatus==0]
          (junction 269) -> (junction 268) [order 2] : [ClawStatus==1]
          (junction 268) -> OpenMax [order 1] : [PWM>=1680]
          (junction 268) -> OpenClaw [order 2] : [PWM<1680]
          (junction 266) -> CloseClaw [order 2] : [PWM>1180]
          (junction 266) -> CloseMax [order 1] : [PWM<=1180]
          (default) -> (junction 269)
        state CheckLEFTY
          state YCenter
            en:
            FrontBack=FrontBack+0;
            LYC=0;
            LHRH = 2;
          state YFront
            en:
            FrontBack=FrontBack-0.02;
            LHRH = 2;
          state YBack
            en:
            FrontBack=FrontBack+0.02;
            LHRH = 2;
          (default) -> (junction 258)
          (junction 258) -> YFront [order 3] : [LeftHand[1]==1]
          (junction 258) -> YCenter [order 2] : [LeftHand[1]==0]
          (junction 258) -> YBack [order 1] : [LeftHand[1]== -1]
        CheckLEFTX -> CheckLEFTY : [(LHRH==1)]
        CheckLEFTY -> CheckLEFTZ : [(LHRH==2)]
        (junction 263) -> CheckLEFTX [order 2] : [LeftHand[2]~= -2]
        CheckLEFTZ -> CheckRIGHTXY : [(LHRH==3)]
        (junction 263) -> CheckRIGHTXY [order 1] : [LeftHand[2]== -2]
        CheckRIGHTXY -> CLAW : [LHRH ==4]
      state Constraint
        state PositionConstraint
          state Xpositive
            en:
            LeftRight=-1;
          state Xnegative
            en:
            LeftRight=-2;
          state Ypositive
            en:
            FrontBack=2;
          state Ynegative
            en:
            FrontBack=-2;
          state Zpositive
            en:
            UpDown=0.78;
          state Znegative
            en:
            UpDown=-1;
          state RotateACW
            en:
            Rotation=-3.1;
          state RotateCW
            en:
            Rotation=3.1;
          state Contained
            en:
            LHRH = 7;
          (junction 260) -> Contained [order 1] : [Rotation>=-3.1]
          Znegative -> (junction 270)
          (default) -> (junction 262)
          (junction 262) -> Xpositive [order 2] : [LeftRight>-1]
          (junction 261) -> Xnegative [order 2] : [LeftRight<-2]
          (junction 275) -> Ypositive [order 2] : [FrontBack>2]
          (junction 274) -> Ynegative [order 2] : [FrontBack<-2]
          (junction 273) -> Zpositive [order 2] : [UpDown>0.78]
          Xnegative -> (junction 275)
          (junction 273) -> (junction 264) [order 1] : [UpDown<=0.78]
          Ypositive -> (junction 274)
          (junction 274) -> (junction 273) [order 1] : [FrontBack>=-2]
          (junction 264) -> (junction 270) [order 1] : [UpDown>=-1]
          RotateACW -> Contained
          RotateCW -> (junction 260)
          (junction 260) -> RotateACW [order 2] : [Rotation<-3.1]
          (junction 270) -> (junction 260) [order 1] : [Rotation<=3.1]
          (junction 270) -> RotateCW [order 2] : [Rotation>3.1]
          Ynegative -> (junction 273)
          Zpositive -> (junction 264)
          (junction 264) -> Znegative [order 2] : [UpDown<-1]
          (junction 262) -> (junction 261) [order 1] : [LeftRight<=-1]
          Xpositive -> (junction 261)
          (junction 261) -> (junction 275) [order 1] : [LeftRight>=-2]
          (junction 275) -> (junction 274) [order 1] : [FrontBack<=2]
        state ALLGreen
          en:
          LHRH = 7;
        (junction 276) -> PositionConstraint [order 2] : [(LeftRight > -1)|(LeftRight<-2)|(FrontBack>2)|(FrontBack<-2)|(UpDown>0.78)|(UpDown<-1)|(Rotation>3.1)|(Rotation<-3.1)]
        (junction 276) -> ALLGreen [order 1] : [(LeftRight<=-1)&(LeftRight>=-2)&(FrontBack<=2)&(FrontBack>=-2)&(UpDown<=0.78)&(UpDown>=-1)&(Rotation<=3.1)&(Rotation>=-3.1)]
        PositionConstraint -> ALLGreen : [(LeftRight<=-1)&(LeftRight>=-2)&(FrontBack<=2)&(FrontBack>=-2)&(UpDown<=0.78)&(UpDown>=-1)&(Rotation<=3.1)&(Rotation>=-3.1)]
        (default) -> (junction 276)
      state CheckKinect
        en:
        PosDesired[0]=-1.5+LeftRight, PosDesired[1]=0+FrontBack,PosDesired[2]= -1.5+UpDown,PosDesired[3] = 0+Rotation;
      KinectTrack -> UpdateQuad [order 1] : [KinectTracking==0]
      (default) -> KinectTrack [order 1] : [KinectTracking==1]
      KinectTrack -> Constraint [order 2] : [(LHRH==5)]
      (default) -> Initialise [order 2]
      Initialise -> UpdateQuad : after (3,sec)
      Constraint -> UpdateQuad : [LHRH==7]
      UpdateQuad -> CheckKinect : [KinectTracking~=1]
      CheckKinect -> UpdateQuad : after (0.2,sec)
    state Safety
      state Descent1
        descentrate=descentrate+0.02;
      state Descent
        en:PosDesired[0] = PerchPos[0]; PosDesired[1] = PerchPos[1];PosDesired[2] = PerchPos[2]-0.50+descentrate;
      state Prelanding
        en:PosDesired[0] = PerchPos[0]; PosDesired[1] = PerchPos[1];PosDesired[2] = PerchPos[2]-0.8 ;
        descentrate=0;
      state SafyHover
        en:PosDesired = Pos; PosDesired[2]= -1.5;
      (default) -> SafyHover
      Descent1 -> Descent : after (0.5,sec)
      Descent -> Descent1 [order 2] : [PerchError < 0.02]
      Descent -> Prelanding [order 1] : after (5,sec)
      Prelanding -> Descent : [PerchError < 0.01]
      SafyHover -> Prelanding : after (3, sec)
    (default) -> TakeOff : {PosDesired = Pos;  PosDesired[2] =-1.2;}
    TakeOff -> Kinect [order 1] : after (7,sec)
    TakeOff -> Safety [order 2] : [RC[5] > 0.5]
    Kinect -> Safety : [RC[5] > 0.5]
  (default) -> Landing : {HoverThrottle = 0;}
  AirBorne -> Landing : [RC[6] < -0.5]
  Landing -> AirBorne : [RC[6] > 0.5]
  data: PosDesired output double size=4; HoverThrottle output double size=1; Mode output uint8 size=1; RC input double size=8; Pos input double size=4; PerchPos input double size=4; DeltaT parameter double size=1; H0 parameter double size=1; Kl parameter double size=1; VelCmd local double size=2 =0; PWM output double; PerchError input double; PI parameter double size=1; descentrate local double; LeftHand input double; KinectTracking input double; UpDown local double; FrontBack local double; XYZchecker local double; RightHand input double; ClawStatus local double; LHRH local double; Rotation local double; LeftRight local double; LXC local double; LYC local double; LZC local double; RXYC local double; safechecker local double; Toggle local double
